simulink model "chap7_10sim"  (Simulink 5.0)
settings: Solver=ode45  StartTime=0.0  StopTime=20  FixedStep=0.001
settings Model: LastModifiedBy=Administrator  AlgebraicLoopMsg=none

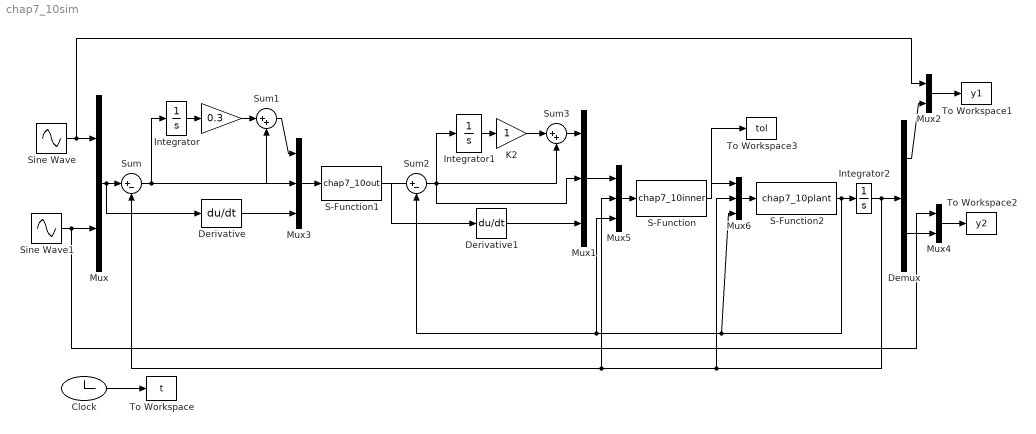
== system chap7_10sim ==
  " " : Gain  Gain=0.3  SaturateOnIntegerOverflow=on
  Clock : Clock
  Demux : Demux  Outputs=2
  Derivative : Derivative
  Derivative1 : Derivative
  Integrator : Integrator
  Integrator1 : Integrator
  Integrator2 : Integrator
  K2 : Gain  SaturateOnIntegerOverflow=on
  Mux : Mux  Inputs=2
  Mux{1,3,5..6} (4 alike) : Mux  Inputs=3
  Mux2 : Mux  Inputs=2
  Mux4 : Mux  Inputs=2
  S-Function : S-Function  FunctionName=chap7_10inner
  S-Function1 : S-Function  FunctionName=chap7_10out
  S-Function2 : S-Function  FunctionName=chap7_10plant
  Sine Wave : Sin  Phase=pi/2  SampleTime=0
  Sine Wave1 : Sin  Phase=pi/2  SampleTime=0
  Sum : Sum  Inputs=|+-  SaturateOnIntegerOverflow=on
  Sum1 : Sum  Inputs=|++  SaturateOnIntegerOverflow=on
  Sum2 : Sum  Inputs=|+-  SaturateOnIntegerOverflow=on
  Sum3 : Sum  Inputs=|++  SaturateOnIntegerOverflow=on  InputSameDT=on
  To Workspace : ToWorkspace  VariableName=t  SampleTime=-1  SaveFormat=Array
  To Workspace1 : ToWorkspace  VariableName=y1  SampleTime=-1  SaveFormat=Array
  To Workspace2 : ToWorkspace  VariableName=y2  SampleTime=-1  SaveFormat=Array
  To Workspace3 : ToWorkspace  VariableName=tol  SampleTime=-1  SaveFormat=Array
  wires:
  S-Function2/1 -> Integrator2/1, Mux6/3, Mux5/3, Sum2/2
  Sine Wave/1 -> Mux/1, Mux2/1
  Integrator2/1 -> Demux/1, Sum/2, Mux5/2, Mux6/2
  Sum/1 -> Integrator/1, Sum1/2, Mux3/2
  Integrator/1 -> " "/1
  " "/1 -> Sum1/1
  Sum1/1 -> Mux3/1
  Derivative/1 -> Mux3/3
  Mux3/1 -> S-Function1/1
  S-Function1/1 -> Derivative1/1, Sum2/1
  Sum2/1 -> Integrator1/1, Sum3/2, Mux1/2
  Integrator1/1 -> K2/1
  K2/1 -> Sum3/1
  Sum3/1 -> Mux1/1
  Derivative1/1 -> Mux1/3
  Mux/1 -> Sum/1, Derivative/1
  Sine Wave1/1 -> Mux4/1, Mux/2
  Demux/1 -> Mux2/2
  Mux2/1 -> To Workspace1/1
  Mux4/1 -> To Workspace2/1
  Demux/2 -> Mux4/2
  Mux5/1 -> S-Function/1
  Mux6/1 -> S-Function2/1
  S-Function/1 -> Mux6/1, To Workspace3/1
  Clock/1 -> To Workspace/1
  Mux1/1 -> Mux5/1
